simulink model "yixiang"  (R2024a)
settings: Solver=FixedStepDiscrete  StartTime=0.0  StopTime=0.01  FixedStep=1e-8  RelTol=1e-3
libraries: hdlsllib x60, simulink x1
(part 1 of 2)
settings Model: Creator=17862  LastModifiedBy=zyy
settings SolverCC: AlgebraicLoopSolver=TrustRegion  AutoInsertRateTranBlk=on
settings DataIOCC: ReturnWorkspaceOutputs=off
settings OptimizationCC: BlockReduction=off  ConditionallyExecuteInputs=off  DefaultParameterBehavior=Inlined
settings DebuggingCC: AlgebraicLoopMsg=error  SingleTaskRateTransMsg=error  UnconnectedInputMsg=warning  UnconnectedOutputMsg=warning  UnconnectedLineMsg=warning  ArithmeticOperatorsInVariantConditions=warning
settings HardwareCC: ProdBitPerPointer=32  ProdBitPerSizeT=32  ProdBitPerPtrDiffT=32  ProdLargestAtomicFloat=None  ProdIntDivRoundTo=Undefined  ProdEndianess=Unspecified  ProdWordSize=32  ProdHWDeviceType=ASIC/FPGA->ASIC/FPGA  TargetBitPerPointer=64  TargetBitPerSizeT=64  TargetBitPerPtrDiffT=64  TargetLongLongMode=on  TargetIntDivRoundTo=Zero  TargetEndianess=LittleEndian  TargetWordSize=64  TargetHWDeviceType=Custom Processor->MATLAB Host Computer  ProdEqTarget=off
settings ModelReferenceCC: EnableRefExpFcnMdlSchedulingChecks=on
settings SFSimCC: CustomCodeUndefinedFunction=UseInterfaceOnly
settings RTWCC: GPUComputeCapability=3.5

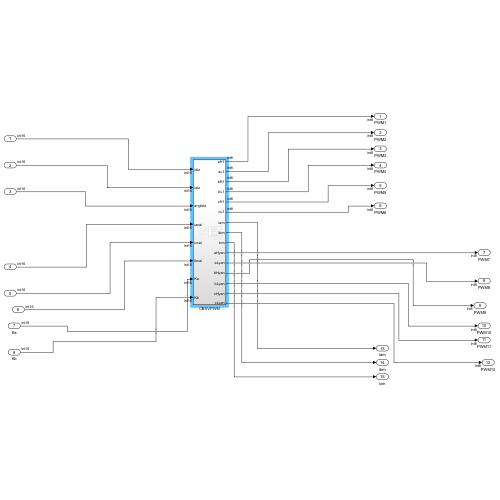
[thumbnail: Simulink's stored preview of the top-level diagram]
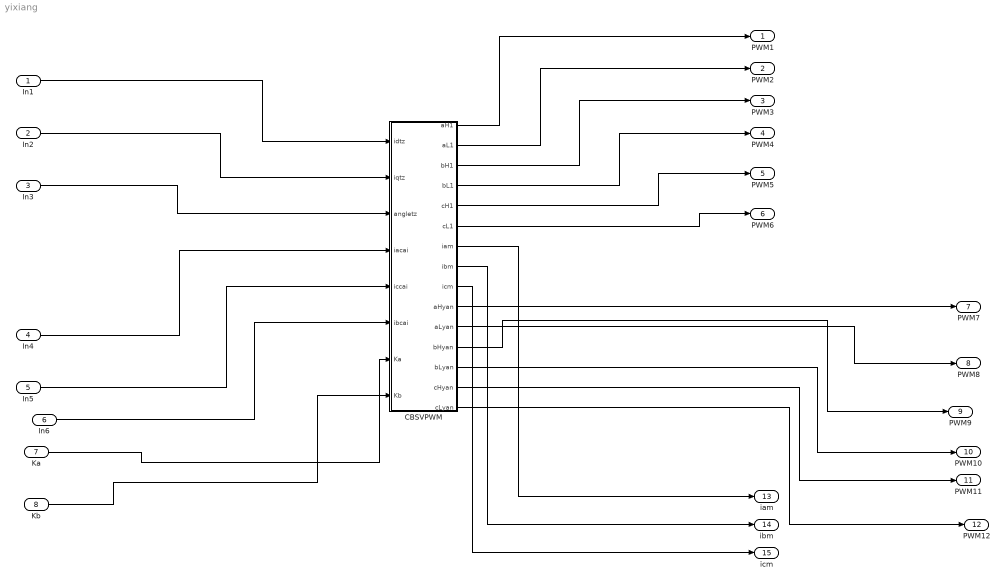
== system yixiang ==
  In1 : Inport  OutDataTypeStr=int16
  In2 : Inport  Port=2  OutDataTypeStr=int16
  In3 : Inport  Port=3  OutDataTypeStr=int16
  In4 : Inport  Port=4  OutDataTypeStr=int16
  In5 : Inport  Port=5  OutDataTypeStr=int16
  In6 : Inport  Port=6  OutDataTypeStr=int16
  Ka : Inport  Port=7  OutDataTypeStr=int16
  Kb : Inport  Port=8  OutDataTypeStr=int16
  CBSVPWM : Subsystem
  PWM1 : Outport  OutDataTypeStr=int8
  PWM2 : Outport  Port=2  OutDataTypeStr=int8
  PWM3 : Outport  Port=3  OutDataTypeStr=int8
  PWM4 : Outport  Port=4  OutDataTypeStr=int8
  PWM5 : Outport  Port=5  OutDataTypeStr=int8
  PWM6 : Outport  Port=6  OutDataTypeStr=int8
  PWM7 : Outport  Port=7  OutDataTypeStr=int8
  PWM8 : Outport  Port=8  OutDataTypeStr=int8
  PWM9 : Outport  Port=9  OutDataTypeStr=int8
  PWM10 : Outport  Port=10  OutDataTypeStr=int8
  PWM11 : Outport  Port=11  OutDataTypeStr=int8
  PWM12 : Outport  Port=12  OutDataTypeStr=int8
  iam : Outport  Port=13
  ibm : Outport  Port=14
  icm : Outport  Port=15
  wires:
  CBSVPWM/12(bHyan) -> PWM9/1
  CBSVPWM/13(bLyan) -> PWM10/1
  CBSVPWM/11(aLyan) -> PWM8/1
  CBSVPWM/15(cLyan) -> PWM12/1
  CBSVPWM/14(cHyan) -> PWM11/1
  CBSVPWM/10(aHyan) -> PWM7/1
  CBSVPWM/6(cL1) -> PWM6/1
  CBSVPWM/5(cH1) -> PWM5/1
  CBSVPWM/2(aL1) -> PWM2/1
  CBSVPWM/1(aH1) -> PWM1/1
  CBSVPWM/3(bH1) -> PWM3/1
  CBSVPWM/4(bL1) -> PWM4/1
  In1/1 -> CBSVPWM/1(idtz)
  In2/1 -> CBSVPWM/2(iqtz)
  In3/1 -> CBSVPWM/3(angletz)
  In4/1 -> CBSVPWM/4(iacai)
  In5/1 -> CBSVPWM/5(iccai)
  In6/1 -> CBSVPWM/6(ibcai)
  CBSVPWM/7(iam) -> iam/1
  CBSVPWM/8(ibm) -> ibm/1
  CBSVPWM/9(icm) -> icm/1
  Ka/1 -> CBSVPWM/7(Ka)
  Kb/1 -> CBSVPWM/8(Kb)

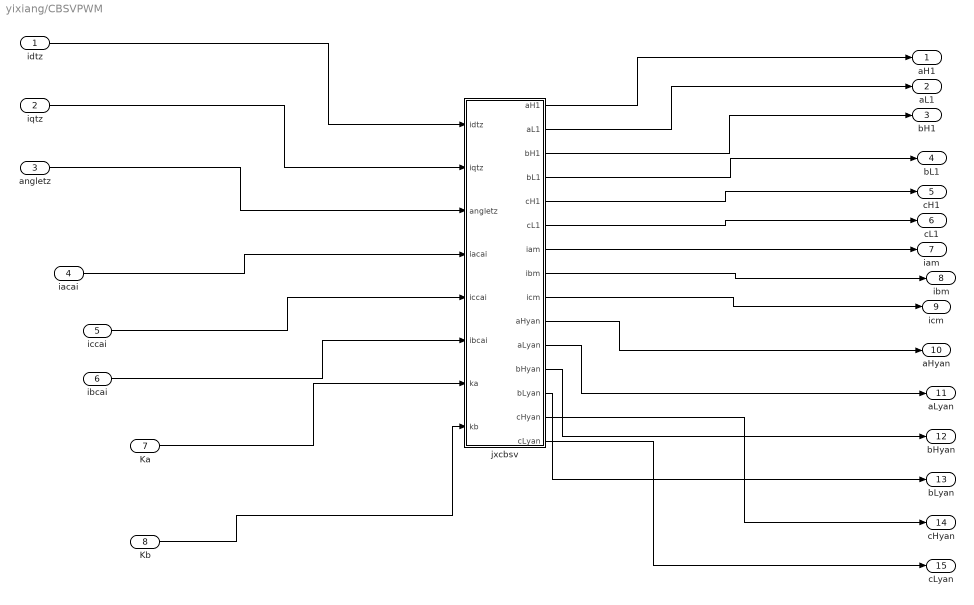
== system yixiang/CBSVPWM ==
  idtz : Inport  OutDataTypeStr=int16
  iqtz : Inport  Port=2  OutDataTypeStr=int16
  angletz : Inport  Port=3  OutDataTypeStr=int16
  iacai : Inport  Port=4  OutDataTypeStr=int16
  iccai : Inport  Port=5  OutDataTypeStr=int16
  ibcai : Inport  Port=6  OutDataTypeStr=int16
  Ka : Inport  Port=7  OutDataTypeStr=int16
  Kb : Inport  Port=8  OutDataTypeStr=int16
  jxcbsv : Subsystem
  aH1 : Outport  OutDataTypeStr=int8
  aL1 : Outport  Port=2  OutDataTypeStr=int8
  bH1 : Outport  Port=3  OutDataTypeStr=int8
  bL1 : Outport  Port=4  OutDataTypeStr=int8
  cH1 : Outport  Port=5  OutDataTypeStr=int8
  cL1 : Outport  Port=6  OutDataTypeStr=int8
  iam : Outport  Port=7
  ibm : Outport  Port=8
  icm : Outport  Port=9
  aHyan : Outport  Port=10
  aLyan : Outport  Port=11
  bHyan : Outport  Port=12
  bLyan : Outport  Port=13
  cHyan : Outport  Port=14
  cLyan : Outport  Port=15
  wires:
  iqtz/1 -> jxcbsv/2(iqtz)
  jxcbsv/6(cL1) -> cL1/1
  jxcbsv/3(bH1) -> bH1/1
  jxcbsv/2(aL1) -> aL1/1
  jxcbsv/4(bL1) -> bL1/1
  iacai/1 -> jxcbsv/4(iacai)
  jxcbsv/5(cH1) -> cH1/1
  jxcbsv/1(aH1) -> aH1/1
  angletz/1 -> jxcbsv/3(angletz)
  idtz/1 -> jxcbsv/1(idtz)
  iccai/1 -> jxcbsv/5(iccai)
  ibcai/1 -> jxcbsv/6(ibcai)
  jxcbsv/7(iam) -> iam/1
  jxcbsv/8(ibm) -> ibm/1
  jxcbsv/9(icm) -> icm/1
  jxcbsv/13(bLyan) -> bLyan/1
  jxcbsv/12(bHyan) -> bHyan/1
  jxcbsv/10(aHyan) -> aHyan/1
  jxcbsv/15(cLyan) -> cLyan/1
  jxcbsv/14(cHyan) -> cHyan/1
  jxcbsv/11(aLyan) -> aLyan/1
  Ka/1 -> jxcbsv/7(ka)
  Kb/1 -> jxcbsv/8(kb)

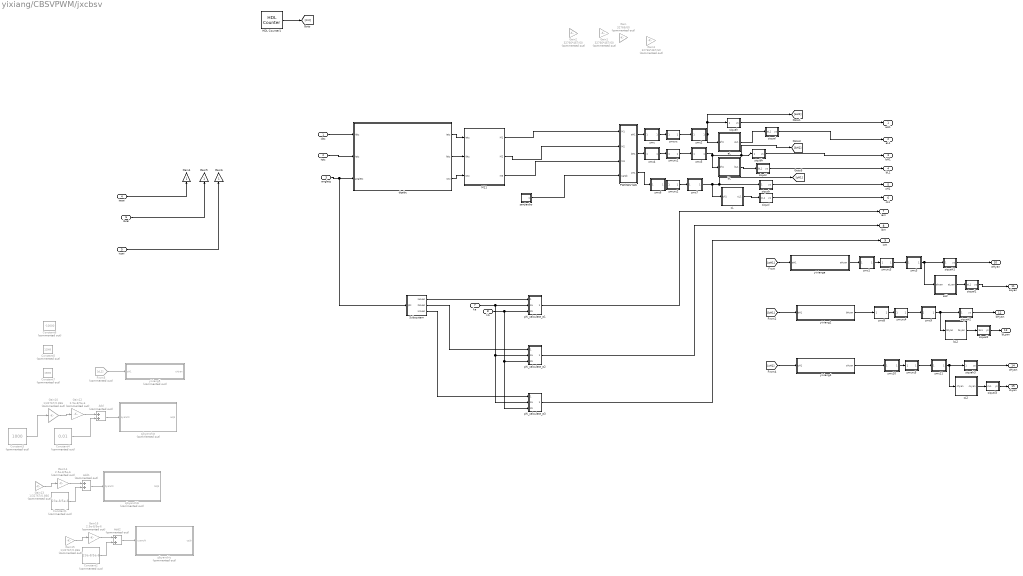
== system yixiang/CBSVPWM/jxcbsv ==
  idtz : Inport  OutDataTypeStr=int16
  iqtz : Inport  Port=2  OutDataTypeStr=int16
  angletz : Inport  Port=3  OutDataTypeStr=int16
  iacai : Inport  Port=4
  iccai : Inport  Port=5
  ibcai : Inport  Port=6
  ka : Inport  Port=7
  kb : Inport  Port=8
  Add : Sum  Commented=on  AccumDataTypeStr=fixdt(1,30,29)
  Add1 : Sum  Commented=on  OutDataTypeStr=fixdt(1,30,29)  AccumDataTypeStr=fixdt(1,30,29)
  Add2 : Sum  Commented=on  OutDataTypeStr=fixdt(1,30,29)  AccumDataTypeStr=fixdt(1,30,29)
  Constant1 : Constant  Commented=on  Value=23e-8/5e-6  OutDataTypeStr=fixdt(1,7,6)  SampleTime=1e-8
  Constant2 : Constant  Commented=on  Value=23e-8/5e-6  OutDataTypeStr=fixdt(1,7,6)  SampleTime=1e-8
  Constant3 : Constant  Commented=on  Value=1000  OutDataTypeStr=int16  SampleTime=1e-8
  Constant4 : Constant  Commented=on  Value=0.01  OutDataTypeStr=fixdt(1,7,6)  SampleTime=1e-8
  Constant5 : Constant  Commented=on  Value=12000  OutDataTypeStr=int16  SampleTime=2e-8
  Constant6 : Constant  Commented=on  Value=-10000  OutDataTypeStr=int16  SampleTime=2e-8
  Constant7 : Constant  Commented=on  Value=15000  OutDataTypeStr=int16  SampleTime=2e-8
  From5 : From  Commented=on  GotoTag=cL1
  Gain : Gain  Commented=on  Gain=32766/60  OutDataTypeStr=int16
  Gain1 : Gain  Commented=on  Gain=32766*4E7/60  OutDataTypeStr=int16
  Gain10 : Gain  Commented=on  Gain=1/32767/0.866  OutDataTypeStr=fixdt(1,21,20)
  Gain12 : Gain  Commented=on  Gain=2.5e-8/5e-6  OutDataTypeStr=fixdt(1,30,29)
  Gain13 : Gain  Commented=on  Gain=1/32767/0.866  OutDataTypeStr=fixdt(1,21,20)
  Gain14 : Gain  Commented=on  Gain=2.5e-8/5e-6  OutDataTypeStr=fixdt(1,30,29)
  Gain15 : Gain  Commented=on  Gain=1/32767/0.866  OutDataTypeStr=fixdt(1,21,20)
  Gain16 : Gain  Commented=on  Gain=2.5e-8/5e-6  OutDataTypeStr=fixdt(1,30,29)
  Gain2 : Gain  Commented=on  Gain=32766*4E7/60  OutDataTypeStr=int16
  Gain3 : Gain  Commented=on  Gain=32766*4E7/60  OutDataTypeStr=int16
  Gain4 : Gain  OutDataTypeStr=int16
  Gain5 : Gain  OutDataTypeStr=int16
  Gain6 : Gain  OutDataTypeStr=int16
  HDL Counter1 : hdlsllib/Sources/HDL Counter  CountType=Count limited  CountInit=0  CountStep=1  CountMax=250  CountFromType=Initial value  CountFrom=0  CountResetPort=off  CountLoadPort=off  CountEnbPort=off  CountDirPort=off  CountHitOutputPort=off  CountDataType=Unsigned  CountWordLen=20  CountFracLen=0  CountSampTime=1/10000/5000
  M11 : Subsystem
  PWMWUYAN : Subsystem
  Subsystem : Subsystem
  aL : Subsystem
  aL2 : Subsystem
  bL : Subsystem
  bL2 : Subsystem
  cL : Subsystem
  cL2 : Subsystem
  dqabc : Subsystem
  phi_calculate_a1 : Subsystem
  phi_calculate_a2 : Subsystem
  phi_calculate_a3 : Subsystem
  sanjiaobo : Subsystem
  siquah : Subsystem
  siquah1 : Subsystem
  siquah2 : Subsystem
  siquah3 : Subsystem
  siqual : Subsystem
  siqual1 : Subsystem
  siqual2 : Subsystem
  siqual3 : Subsystem
  siqubh : Subsystem
  siqubl : Subsystem
  siquch : Subsystem
  siqucl : Subsystem
  sjbyanchia : Subsystem  Commented=on
  sjbyanchib : Subsystem  Commented=on
  sjbyanchic : Subsystem  Commented=on
  yixiang2 : Subsystem
  yixiang4 : Subsystem
  yixiang5 : Subsystem  Commented=on
  yixianga : Subsystem
  zmc : Subsystem
  zmc1 : Subsystem
  zmc10 : Subsystem
  zmc11 : Subsystem
  zmc2 : Subsystem
  zmc3 : Subsystem
  zmc4 : Subsystem
  zmc5 : Subsystem
  zmc6 : Subsystem
  zmc7 : Subsystem
  zmc8 : Subsystem
  zmc9 : Subsystem
  zmcxc : Subsystem
  zmcxc1 : Subsystem
  zmcxc2 : Subsystem
  zmcxc3 : Subsystem
  zmcxc4 : Subsystem
  zmcxc5 : Subsystem
  aH1 : Outport  OutDataTypeStr=int8
  aL1 : Outport  Port=2  OutDataTypeStr=int8
  bH1 : Outport  Port=3  OutDataTypeStr=int8
  bL1 : Outport  Port=4  OutDataTypeStr=int8
  cH1 : Outport  Port=5  OutDataTypeStr=int8
  cL1 : Outport  Port=6  OutDataTypeStr=int8
  iam : Outport  Port=7
  ibm : Outport  Port=8
  icm : Outport  Port=9
  aHyan : Outport  Port=10  OutDataTypeStr=int8
  aLyan : Outport  Port=11  OutDataTypeStr=int8
  bHyan : Outport  Port=12  OutDataTypeStr=int8
  bLyan : Outport  Port=13  OutDataTypeStr=int8
  cHyan : Outport  Port=14  OutDataTypeStr=int8
  cLyan : Outport  Port=15  OutDataTypeStr=int8
  wires:
  iqtz/1 -> dqabc/2(iqtz)
  idtz/1 -> dqabc/1(idtz)
  dqabc/1(iatz) -> M11/1(iatz)
  dqabc/2(ibtz) -> M11/2(ibtz)
  dqabc/3(ictz) -> M11/3(ictz)
  Add/1 -> sjbyanchia/1(ayanchi)
  Gain12/1 -> Add/1
  Gain10/1 -> Gain12/1
  sanjiaobo/1(sanjb) -> PWMWUYAN/4(sanjb)
  Add2/1 -> sjbyanchic/1(cyanchi)
  Gain15/1 -> Gain16/1
  Gain16/1 -> Add2/1
  Constant2/1 -> Add2/2
  Add1/1 -> sjbyanchib/1(byanchi)
  Gain13/1 -> Gain14/1
  Gain14/1 -> Add1/1
  Constant1/1 -> Add1/2
  Constant4/1 -> Add/2
  Constant3/1 -> Gain10/1
  HDL Counter1/1 -> [cnt]
  M11/2(M2) -> PWMWUYAN/2(M2)
  M11/3(M3) -> PWMWUYAN/3(M3)
  M11/1(M1) -> PWMWUYAN/1(M1)
  PWMWUYAN/1(aH1) -> zmc/1(aH1)
  zmc/1(bH1) -> zmcxc/1(bH1)
  zmcxc/1(aL1) -> zmc2/1(aH1)
  zmc2/1(bH1) -> siquah/1(aH1), [aH1], aL/1(ah1)
  zmc4/1(bH1) -> zmcxc1/1(bH1)
  zmcxc1/1(aL1) -> zmc5/1(aH1)
  aL/1(aL1) -> siqual/1(aL1)
  PWMWUYAN/2(bH1) -> zmc4/1(aH1)
  zmc5/1(bH1) -> bL/1(bh1), [bH1], siqubh/1(bH1)
  bL/1(bL1) -> siqubl/1(bL1)
  zmc6/1(bH1) -> zmcxc2/1(bH1)
  zmcxc2/1(aL1) -> zmc7/1(aH1)
  PWMWUYAN/3(cH1) -> zmc6/1(aH1)
  zmc7/1(bH1) -> [cH1], siquch/1(cH1), cL/1(ch1)
  cL/1(cL1) -> siqucl/1(cL1)
  siqubl/1(ys) -> bL1/1
  siquah/1(ys) -> aH1/1
  siqubh/1(ys) -> bH1/1
  siquch/1(ys) -> cH1/1
  siqucl/1(ys) -> cL1/1
  iacai/1 -> Gain4/1
  ibcai/1 -> Gain5/1
  iccai/1 -> Gain6/1
  phi_calculate_a1/1(iam) -> iam/1
  angletz/1 -> Subsystem/1(phi), dqabc/3(angletz)
  Subsystem/1(iasuan) -> phi_calculate_a1/1(iacai)
  ka/1 -> phi_calculate_a3/2(ka), phi_calculate_a2/2(ka), phi_calculate_a1/2(ka)
  kb/1 -> phi_calculate_a3/3(kb), phi_calculate_a2/3(kb), phi_calculate_a1/3(kb)
  siqual/1(ys) -> aL1/1
  [aH1] -> yixianga/1(aH1)
  [bH1] -> yixiang2/1(bH1)
  [cH1] -> yixiang4/1(cH1)
  From5/1 -> yixiang5/1(cH1)
  Subsystem/2(ibsuan) -> phi_calculate_a2/1(ibcai)
  Subsystem/3(icsuan) -> phi_calculate_a3/1(iccai)
  phi_calculate_a2/1(ibm) -> ibm/1
  phi_calculate_a3/1(icm) -> icm/1
  aL2/1(aLyan) -> siqual1/1(aL1)
  yixianga/1(aHyan) -> zmc1/1(aH1)
  zmc3/1(bH1) -> aL2/1(ahyan), siquah1/1(aH1)
  zmcxc3/1(aL1) -> zmc3/1(aH1)
  zmc1/1(bH1) -> zmcxc3/1(bH1)
  zmcxc4/1(aL1) -> zmc9/1(aH1)
  yixiang2/1(bHyan) -> zmc8/1(aH1)
  zmc8/1(bH1) -> zmcxc4/1(bH1)
  zmc9/1(bH1) -> bL2/1(bhyan), siquah2/1(bH1)
  siqual1/1(ys) -> aLyan/1
  siquah1/1(ys) -> aHyan/1
  siquah2/1(ys) -> bHyan/1
  siqual2/1(ys) -> bLyan/1
  bL2/1(bLyan) -> siqual2/1(bL1)
  zmc10/1(bH1) -> zmcxc5/1(bH1)
  zmcxc5/1(aL1) -> zmc11/1(aH1)
  yixiang4/1(cHyan) -> zmc10/1(aH1)
  zmc11/1(bH1) -> cL2/1(chyan), siquah3/1(cH1)
  cL2/1(cLyan) -> siqual3/1(cL1)
  siquah3/1(ys) -> cHyan/1
  siqual3/1(ys) -> cLyan/1

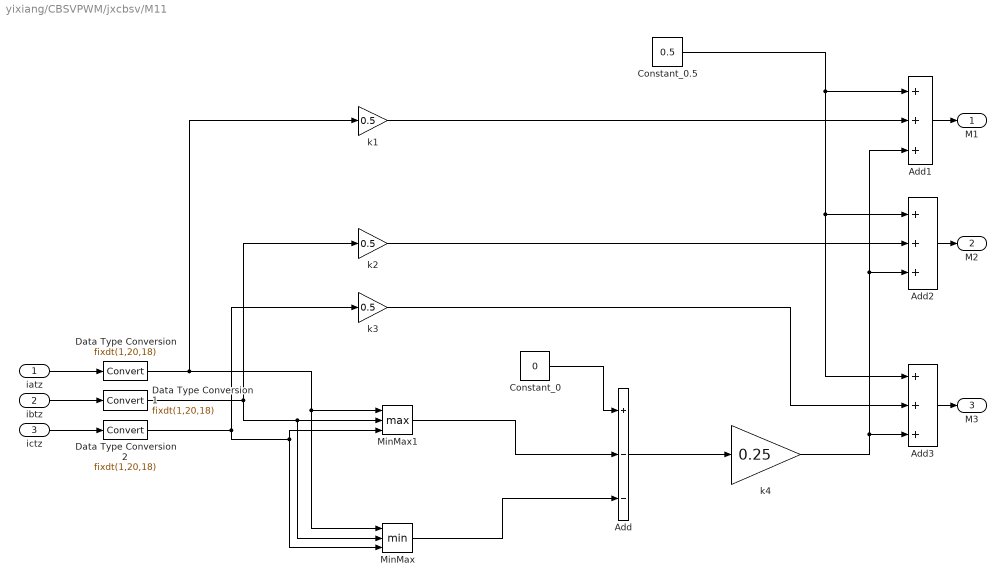
== system yixiang/CBSVPWM/jxcbsv/M11 ==
  iatz : Inport
  ibtz : Inport  Port=2
  ictz : Inport  Port=3
  Add : Sum  Inputs=+--  OutDataTypeStr=fixdt(1,20,18)
  Add1 : Sum  Inputs=+++  OutDataTypeStr=fixdt(1,20,18)  AccumDataTypeStr=fixdt(1,20,18)
  Add2 : Sum  Inputs=+++  OutDataTypeStr=fixdt(1,20,18)  AccumDataTypeStr=fixdt(1,20,18)
  Add3 : Sum  Inputs=+++  OutDataTypeStr=fixdt(1,20,18)  AccumDataTypeStr=fixdt(1,20,18)
  Constant_0 : Constant  Value=0  OutDataTypeStr=fixdt(1,20,18)  SampleTime=2e-8
  Constant_0.5 : Constant  Value=0.5  OutDataTypeStr=fixdt(1,20,18)  SampleTime=2e-8
  Data Type Conversion : DataTypeConversion  OutDataTypeStr=fixdt(1,20,18)  SaturateOnIntegerOverflow=off  RndMeth=Floor
  Data Type Conversion1 : DataTypeConversion  OutDataTypeStr=fixdt(1,20,18)  SaturateOnIntegerOverflow=off  RndMeth=Floor
  Data Type Conversion2 : DataTypeConversion  OutDataTypeStr=fixdt(1,20,18)  SaturateOnIntegerOverflow=off  RndMeth=Floor
  MinMax : MinMax  Inputs=3
  MinMax1 : MinMax  Function=max  Inputs=3
  k1 : Gain  Gain=0.5  OutDataTypeStr=fixdt(1,20,18)
  k2 : Gain  Gain=0.5  OutDataTypeStr=fixdt(1,20,18)
  k3 : Gain  Gain=0.5  OutDataTypeStr=fixdt(1,20,18)
  k4 : Gain  Gain=0.25  OutDataTypeStr=fixdt(1,20,18)
  M1 : Outport  VectorParamsAs1DForOutWhenUnconnected=off
  M2 : Outport  Port=2  VectorParamsAs1DForOutWhenUnconnected=off
  M3 : Outport  Port=3  VectorParamsAs1DForOutWhenUnconnected=off
  wires:
  Constant_0/1 -> Add/1
  Add/1 -> k4/1
  MinMax1/1 -> Add/2
  Add1/1 -> M1/1
  Add2/1 -> M2/1
  Add3/1 -> M3/1
  Constant_0.5/1 -> Add3/1, Add2/1, Add1/1
  k1/1 -> Add1/2
  k4/1 -> Add1/3, Add2/3, Add3/3
  k2/1 -> Add2/2
  k3/1 -> Add3/2
  ibtz/1 -> Data Type Conversion1/1
  ictz/1 -> Data Type Conversion2/1
  MinMax/1 -> Add/3
  iatz/1 -> Data Type Conversion/1
  Data Type Conversion1/1 -> k2/1, MinMax1/2, MinMax/2
  Data Type Conversion2/1 -> k3/1, MinMax1/3, MinMax/3
  Data Type Conversion/1 -> MinMax1/1, MinMax/1, k1/1

== system yixiang/CBSVPWM/jxcbsv/PWMWUYAN ==
  M1 : Inport
  M2 : Inport  Port=2
  M3 : Inport  Port=3
  sanjb : Inport  Port=4
  Add : Sum  Inputs=+-
  Add2 : Sum  Inputs=+-
  Add4 : Sum  Inputs=+-
  Relay : Relay  OnSwitchValue=0  OffSwitchValue=0  OutDataTypeStr=int8
  Relay1 : Relay  OnSwitchValue=0  OffSwitchValue=0  OutDataTypeStr=int8
  Relay2 : Relay  OnSwitchValue=0  OffSwitchValue=0  OutDataTypeStr=int8
  aH1 : Outport  VectorParamsAs1DForOutWhenUnconnected=off
  bH1 : Outport  Port=2  VectorParamsAs1DForOutWhenUnconnected=off
  cH1 : Outport  Port=3  VectorParamsAs1DForOutWhenUnconnected=off
  wires:
  M1/1 -> Add/1
  M3/1 -> Add4/1
  M2/1 -> Add2/1
  Add/1 -> Relay/1
  Add4/1 -> Relay2/1
  Add2/1 -> Relay1/1
  sanjb/1 -> Add4/2, Add2/2, Add/2
  Relay/1 -> aH1/1
  Relay1/1 -> bH1/1
  Relay2/1 -> cH1/1

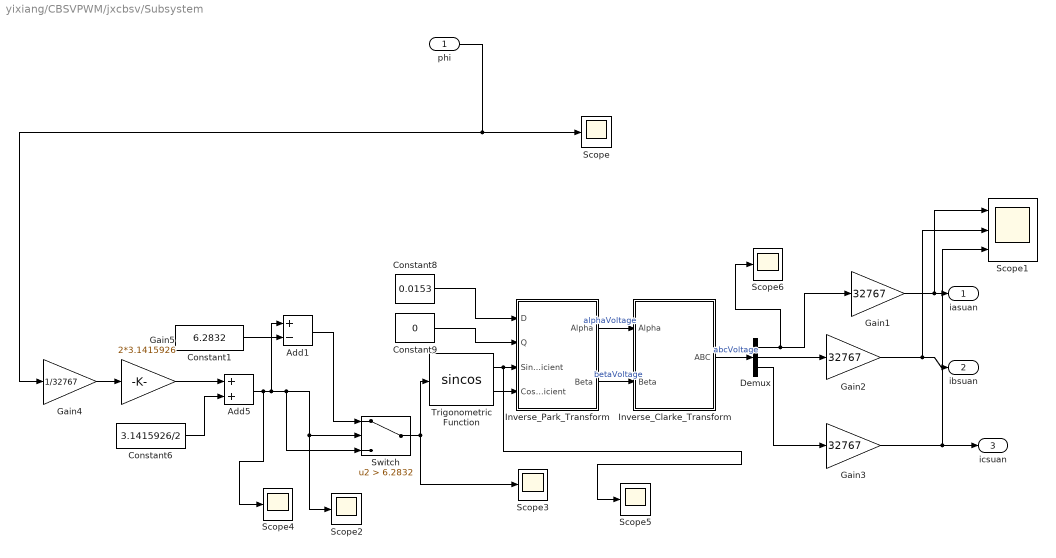
== system yixiang/CBSVPWM/jxcbsv/Subsystem ==
  phi : Inport
  Add1 : Sum  Inputs=+-  OutDataTypeStr=fixdt(1,16,10)  AccumDataTypeStr=fixdt(1,16,10)
  Add5 : Sum  OutDataTypeStr=fixdt(1,16,10)  AccumDataTypeStr=fixdt(1,16,10)
  Constant1 : Constant  Value=6.2832  OutDataTypeStr=fixdt(1,16,10)  SampleTime=2e-8
  Constant6 : Constant  Value=3.1415926/2  OutDataTypeStr=fixdt(1,16,10)  SampleTime=2e-8
  Constant8 : Constant  Value=0.0153  OutDataTypeStr=fixdt(1,32,27)  SampleTime=2e-8
  Constant9 : Constant  Value=0  OutDataTypeStr=uint16  SampleTime=2e-8
  Demux : Demux  Outputs=3
  Gain1 : Gain  Gain=32767  OutDataTypeStr=int16
  Gain2 : Gain  Gain=32767  OutDataTypeStr=int16
  Gain3 : Gain  Gain=32767  OutDataTypeStr=int16
  Gain4 : Gain  Gain=1/32767  OutDataTypeStr=fixdt(1,16,10)
  Gain5 : Gain  Gain=2*3.1415926  OutDataTypeStr=fixdt(1,16,10)
  Inverse_Clarke_Transform : Subsystem  VariantControl=INVERSE_CLARKE_TRANSFORM
      mask Display:
      | port_label('input',1,'\alpha','texmode', 'on')
      | port_label('input',2,'\beta','texmode', 'on')
      | port_label('output',1,'ABC')
  Inverse_Park_Transform : Subsystem
      mask Display:
      | port_label('input',1,'D')
      | port_label('input',2,'Q')
      | port_label('input',3,'Sin')
      | port_label('input',4,'Cos')
      | port_label('output',1,'\alpha','texmode', 'on')
      | port_label('output',2,'\beta','texmode', 'on')
  Scope{,2..6} (6 alike) : Scope
  Scope1 : Scope  NumInputPorts=3
  Switch : Switch  Criteria=u2 > Threshold  Threshold=6.2832  OutDataTypeStr=fixdt(1,16,10)  SaturateOnIntegerOverflow=off  InputSameDT=off
  Trigonometric Function : Trigonometry  Operator=sincos  ApproximationMethod=CORDIC  NumberOfIterations=16
  iasuan : Outport
  ibsuan : Outport  Port=2
  icsuan : Outport  Port=3
  wires:
  Inverse_Park_Transform/1(Alpha) -> Inverse_Clarke_Transform/1(Alpha)  "alphaVoltage"
  Inverse_Clarke_Transform/1(ABC) -> Demux/1  "abcVoltage"
  Inverse_Park_Transform/2(Beta) -> Inverse_Clarke_Transform/2(Beta)  "betaVoltage"
  Constant8/1 -> Inverse_Park_Transform/1(D)
  Constant9/1 -> Inverse_Park_Transform/2(Q)
  Gain4/1 -> Gain5/1
  Trigonometric Function/1 -> Scope5/1, Inverse_Park_Transform/3(Sin_Coefficient)
  Trigonometric Function/2 -> Inverse_Park_Transform/4(Cos_Coefficient)
  Demux/3 -> Gain3/1
  phi/1 -> Scope/1, Gain4/1
  Demux/1 -> Scope6/1, Gain1/1
  Demux/2 -> Gain2/1
  Gain5/1 -> Add5/1
  Add5/1 -> Scope4/1, Add1/1, Switch/3, Scope2/1, Switch/2
  Constant6/1 -> Add5/2
  Gain1/1 -> Scope1/1, iasuan/1
  Gain2/1 -> Scope1/2, ibsuan/1
  Gain3/1 -> Scope1/3, icsuan/1
  Switch/1 -> Trigonometric Function/1, Scope3/1
  Add1/1 -> Switch/1
  Constant1/1 -> Add1/2

== system yixiang/CBSVPWM/jxcbsv/aL ==
  ah1 : Inport
  Data Type Conversion : DataTypeConversion  OutDataTypeStr=boolean  SaturateOnIntegerOverflow=off  RndMeth=Floor
  Data Type Conversion1 : DataTypeConversion  OutDataTypeStr=int8  SaturateOnIntegerOverflow=off  RndMeth=Floor
  Logical Operator : Logic  Operator=NOT  AllPortsSameDT=off  OutDataTypeStr=boolean
  aL1 : Outport  VectorParamsAs1DForOutWhenUnconnected=off
  wires:
  Logical Operator/1 -> Data Type Conversion1/1
  ah1/1 -> Data Type Conversion/1
  Data Type Conversion/1 -> Logical Operator/1
  Data Type Conversion1/1 -> aL1/1

== system yixiang/CBSVPWM/jxcbsv/aL2 ==
  ahyan : Inport
  Data Type Conversion : DataTypeConversion  OutDataTypeStr=boolean  SaturateOnIntegerOverflow=off  RndMeth=Floor
  Data Type Conversion1 : DataTypeConversion  OutDataTypeStr=int8  SaturateOnIntegerOverflow=off  RndMeth=Floor
  Logical Operator : Logic  Operator=NOT  AllPortsSameDT=off  OutDataTypeStr=boolean
  aLyan : Outport  VectorParamsAs1DForOutWhenUnconnected=off
  wires:
  Logical Operator/1 -> Data Type Conversion1/1
  ahyan/1 -> Data Type Conversion/1
  Data Type Conversion/1 -> Logical Operator/1
  Data Type Conversion1/1 -> aLyan/1

== system yixiang/CBSVPWM/jxcbsv/bL ==
  bh1 : Inport
  Data Type Conversion : DataTypeConversion  OutDataTypeStr=boolean  SaturateOnIntegerOverflow=off  RndMeth=Floor
  Data Type Conversion1 : DataTypeConversion  OutDataTypeStr=int8  SaturateOnIntegerOverflow=off  RndMeth=Floor
  Logical Operator : Logic  Operator=NOT  AllPortsSameDT=off  OutDataTypeStr=boolean
  bL1 : Outport  VectorParamsAs1DForOutWhenUnconnected=off
  wires:
  Data Type Conversion1/1 -> bL1/1
  Logical Operator/1 -> Data Type Conversion1/1
  bh1/1 -> Data Type Conversion/1
  Data Type Conversion/1 -> Logical Operator/1

== system yixiang/CBSVPWM/jxcbsv/bL2 ==
  bhyan : Inport
  Data Type Conversion : DataTypeConversion  OutDataTypeStr=boolean  SaturateOnIntegerOverflow=off  RndMeth=Floor
  Data Type Conversion1 : DataTypeConversion  OutDataTypeStr=int8  SaturateOnIntegerOverflow=off  RndMeth=Floor
  Logical Operator : Logic  Operator=NOT  AllPortsSameDT=off  OutDataTypeStr=boolean
  bLyan : Outport  VectorParamsAs1DForOutWhenUnconnected=off
  wires:
  Logical Operator/1 -> Data Type Conversion1/1
  bhyan/1 -> Data Type Conversion/1
  Data Type Conversion/1 -> Logical Operator/1
  Data Type Conversion1/1 -> bLyan/1

== system yixiang/CBSVPWM/jxcbsv/cL ==
  ch1 : Inport
  Data Type Conversion : DataTypeConversion  OutDataTypeStr=boolean  SaturateOnIntegerOverflow=off  RndMeth=Floor
  Data Type Conversion1 : DataTypeConversion  OutDataTypeStr=int8  SaturateOnIntegerOverflow=off  RndMeth=Floor
  Logical Operator : Logic  Operator=NOT  AllPortsSameDT=off  OutDataTypeStr=boolean
  cL1 : Outport  VectorParamsAs1DForOutWhenUnconnected=off
  wires:
  Data Type Conversion1/1 -> cL1/1
  Logical Operator/1 -> Data Type Conversion1/1
  ch1/1 -> Data Type Conversion/1
  Data Type Conversion/1 -> Logical Operator/1

== system yixiang/CBSVPWM/jxcbsv/cL2 ==
  chyan : Inport
  Data Type Conversion : DataTypeConversion  OutDataTypeStr=boolean  SaturateOnIntegerOverflow=off  RndMeth=Floor
  Data Type Conversion1 : DataTypeConversion  OutDataTypeStr=int8  SaturateOnIntegerOverflow=off  RndMeth=Floor
  Logical Operator : Logic  Operator=NOT  AllPortsSameDT=off  OutDataTypeStr=boolean
  cLyan : Outport  VectorParamsAs1DForOutWhenUnconnected=off
  wires:
  Logical Operator/1 -> Data Type Conversion1/1
  chyan/1 -> Data Type Conversion/1
  Data Type Conversion/1 -> Logical Operator/1
  Data Type Conversion1/1 -> cLyan/1

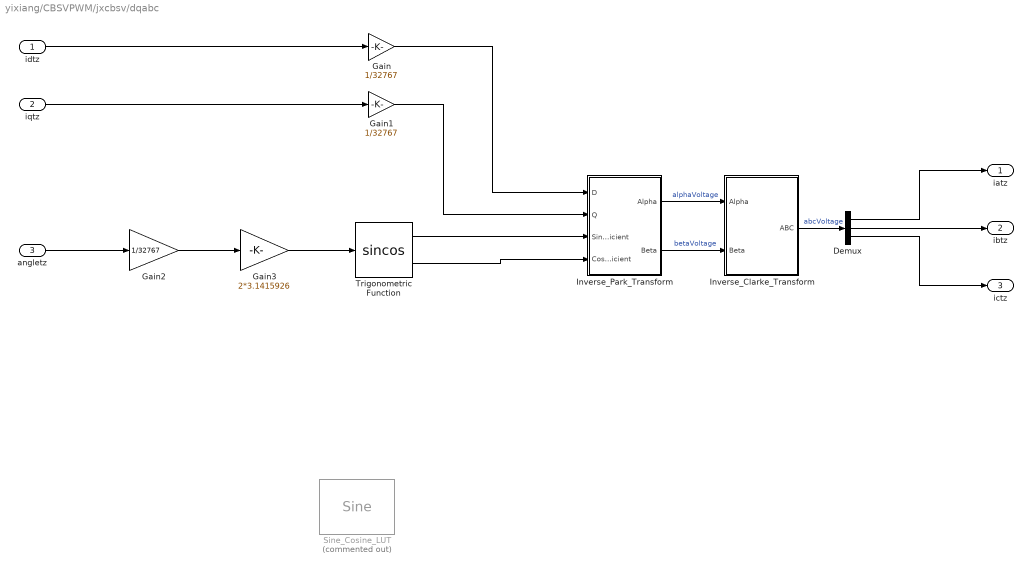
== system yixiang/CBSVPWM/jxcbsv/dqabc ==
  idtz : Inport
  iqtz : Inport  Port=2
  angletz : Inport  Port=3
  Demux : Demux  Outputs=3
  Gain : Gain  Gain=1/32767  OutDataTypeStr=fixdt(1,32,27)
  Gain1 : Gain  Gain=1/32767  OutDataTypeStr=fixdt(1,32,27)
  Gain2 : Gain  Gain=1/32767  OutDataTypeStr=fixdt(1,16,10)
  Gain3 : Gain  Gain=2*3.1415926  OutDataTypeStr=fixdt(1,16,10)
  Inverse_Clarke_Transform : Subsystem  VariantControl=INVERSE_CLARKE_TRANSFORM
      mask Display:
      | port_label('input',1,'\alpha','texmode', 'on')
      | port_label('input',2,'\beta','texmode', 'on')
      | port_label('output',1,'ABC')
  Inverse_Park_Transform : Subsystem
      mask Display:
      | port_label('input',1,'D')
      | port_label('input',2,'Q')
      | port_label('input',3,'Sin')
      | port_label('input',4,'Cos')
      | port_label('output',1,'\alpha','texmode', 'on')
      | port_label('output',2,'\beta','texmode', 'on')
  Sine_Cosine_LUT : simulink/Lookup Tables/Sine  Commented=on  Formula=sin(2*pi*u) and cos(2*pi*u)  NumDataPoints=(2^5)+1  OutputWordLength=32  InternalRulePriority=Speed
  Trigonometric Function : Trigonometry  Operator=sincos  ApproximationMethod=CORDIC  NumberOfIterations=16
  iatz : Outport
  ibtz : Outport  Port=2
  ictz : Outport  Port=3
  wires:
  Gain1/1 -> Inverse_Park_Transform/2(Q)
  Gain/1 -> Inverse_Park_Transform/1(D)
  Inverse_Park_Transform/2(Beta) -> Inverse_Clarke_Transform/2(Beta)  "betaVoltage"
  Inverse_Clarke_Transform/1(ABC) -> Demux/1  "abcVoltage"
  Inverse_Park_Transform/1(Alpha) -> Inverse_Clarke_Transform/1(Alpha)  "alphaVoltage"
  idtz/1 -> Gain/1
  angletz/1 -> Gain2/1
  iqtz/1 -> Gain1/1
  Demux/2 -> ibtz/1
  Demux/1 -> iatz/1
  Trigonometric Function/1 -> Inverse_Park_Transform/3(Sin_Coefficient)
  Trigonometric Function/2 -> Inverse_Park_Transform/4(Cos_Coefficient)
  Gain3/1 -> Trigonometric Function/1
  Gain2/1 -> Gain3/1
  Demux/3 -> ictz/1

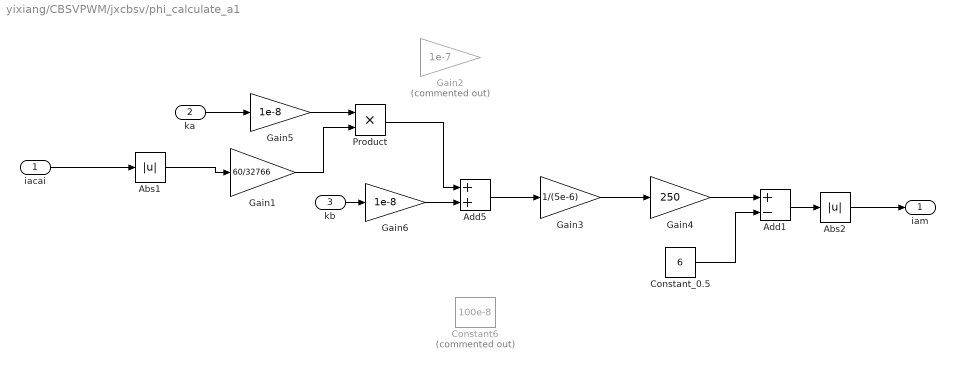
== system yixiang/CBSVPWM/jxcbsv/phi_calculate_a1 ==
  iacai : Inport
  ka : Inport  Port=2
  kb : Inport  Port=3
  Abs1 : Abs  OutDataTypeStr=uint16  SaturateOnIntegerOverflow=off
  Abs2 : Abs  OutDataTypeStr=int16  SaturateOnIntegerOverflow=off
  Add1 : Sum  Inputs=+-  OutDataTypeStr=int16  AccumDataTypeStr=int16
  Add5 : Sum  OutDataTypeStr=fixdt(0,64,40)  AccumDataTypeStr=fixdt(0,64,40)
  Constant6 : Constant  Commented=on  Value=100e-8  OutDataTypeStr=fixdt(0,64,40)  SampleTime=2e-8
  Constant_0.5 : Constant  Value=6  OutDataTypeStr=int16  SampleTime=2e-8
  Gain1 : Gain  Gain=60/32766  OutDataTypeStr=fixdt(0,64,40)
  Gain2 : Gain  Commented=on  Gain=1e-7  OutDataTypeStr=fixdt(0,64,40)
  Gain3 : Gain  Gain=1/(5e-6)  OutDataTypeStr=fixdt(0,64,40)
  Gain4 : Gain  Gain=250  OutDataTypeStr=int16
  Gain5 : Gain  Gain=1e-8  OutDataTypeStr=fixdt(0,64,40)
  Gain6 : Gain  Gain=1e-8  OutDataTypeStr=fixdt(0,64,40)
  Product : Product  OutDataTypeStr=fixdt(0,64,40)
  iam : Outport
  wires:
  Add5/1 -> Gain3/1
  Gain3/1 -> Gain4/1
  iacai/1 -> Abs1/1
  Abs1/1 -> Gain1/1
  Gain4/1 -> Add1/1
  Product/1 -> Add5/1
  Gain1/1 -> Product/2
  ka/1 -> Gain5/1
  kb/1 -> Gain6/1
  Gain5/1 -> Product/1
  Gain6/1 -> Add5/2
  Add1/1 -> Abs2/1
  Abs2/1 -> iam/1
  Constant_0.5/1 -> Add1/2

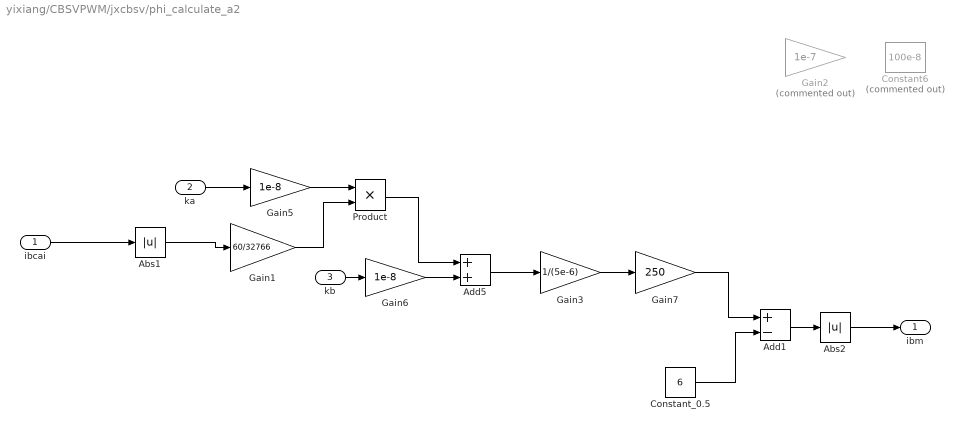
== system yixiang/CBSVPWM/jxcbsv/phi_calculate_a2 ==
  ibcai : Inport
  ka : Inport  Port=2
  kb : Inport  Port=3
  Abs1 : Abs  OutDataTypeStr=uint16  SaturateOnIntegerOverflow=off
  Abs2 : Abs  OutDataTypeStr=int16  SaturateOnIntegerOverflow=off
  Add1 : Sum  Inputs=+-  OutDataTypeStr=int16  AccumDataTypeStr=int16
  Add5 : Sum  OutDataTypeStr=fixdt(0,64,40)  AccumDataTypeStr=fixdt(0,64,40)
  Constant6 : Constant  Commented=on  Value=100e-8  OutDataTypeStr=fixdt(0,64,40)  SampleTime=2e-8
  Constant_0.5 : Constant  Value=6  OutDataTypeStr=int16  SampleTime=2e-8
  Gain1 : Gain  Gain=60/32766  OutDataTypeStr=fixdt(0,64,40)
  Gain2 : Gain  Commented=on  Gain=1e-7  OutDataTypeStr=fixdt(0,64,40)
  Gain3 : Gain  Gain=1/(5e-6)  OutDataTypeStr=fixdt(0,64,40)
  Gain5 : Gain  Gain=1e-8  OutDataTypeStr=fixdt(0,64,40)
  Gain6 : Gain  Gain=1e-8  OutDataTypeStr=fixdt(0,64,40)
  Gain7 : Gain  Gain=250  OutDataTypeStr=int16
  Product : Product  OutDataTypeStr=fixdt(0,64,40)
  ibm : Outport
  wires:
  Add5/1 -> Gain3/1
  Gain3/1 -> Gain7/1
  ibcai/1 -> Abs1/1
  Abs1/1 -> Gain1/1
  Abs2/1 -> ibm/1
  Product/1 -> Add5/1
  Gain1/1 -> Product/2
  ka/1 -> Gain5/1
  kb/1 -> Gain6/1
  Gain5/1 -> Product/1
  Gain6/1 -> Add5/2
  Add1/1 -> Abs2/1
  Gain7/1 -> Add1/1
  Constant_0.5/1 -> Add1/2

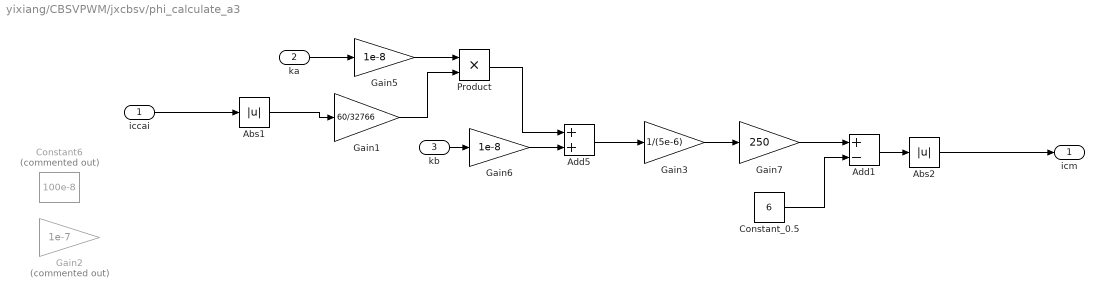
== system yixiang/CBSVPWM/jxcbsv/phi_calculate_a3 ==
  iccai : Inport
  ka : Inport  Port=2
  kb : Inport  Port=3
  Abs1 : Abs  OutDataTypeStr=uint16  SaturateOnIntegerOverflow=off
  Abs2 : Abs  OutDataTypeStr=int16  SaturateOnIntegerOverflow=off
  Add1 : Sum  Inputs=+-  OutDataTypeStr=int16  AccumDataTypeStr=int16
  Add5 : Sum  OutDataTypeStr=fixdt(0,64,40)  AccumDataTypeStr=fixdt(0,64,40)
  Constant6 : Constant  Commented=on  Value=100e-8  OutDataTypeStr=fixdt(0,64,40)  SampleTime=2e-8
  Constant_0.5 : Constant  Value=6  OutDataTypeStr=int16  SampleTime=2e-8
  Gain1 : Gain  Gain=60/32766  OutDataTypeStr=fixdt(0,64,40)
  Gain2 : Gain  Commented=on  Gain=1e-7  OutDataTypeStr=fixdt(0,64,40)
  Gain3 : Gain  Gain=1/(5e-6)  OutDataTypeStr=fixdt(0,64,40)
  Gain5 : Gain  Gain=1e-8  OutDataTypeStr=fixdt(0,64,40)
  Gain6 : Gain  Gain=1e-8  OutDataTypeStr=fixdt(0,64,40)
  Gain7 : Gain  Gain=250  OutDataTypeStr=int16
  Product : Product  OutDataTypeStr=fixdt(0,64,40)
  icm : Outport
  wires:
  Add5/1 -> Gain3/1
  iccai/1 -> Abs1/1
  Abs1/1 -> Gain1/1
  Product/1 -> Add5/1
  Gain1/1 -> Product/2
  ka/1 -> Gain5/1
  kb/1 -> Gain6/1
  Gain5/1 -> Product/1
  Gain6/1 -> Add5/2
  Add1/1 -> Abs2/1
  Gain7/1 -> Add1/1
  Abs2/1 -> icm/1
  Constant_0.5/1 -> Add1/2
  Gain3/1 -> Gain7/1

== system yixiang/CBSVPWM/jxcbsv/sanjiaobo ==
  Abs1 : Abs  OutDataTypeStr=fixdt(1,32,30)  SaturateOnIntegerOverflow=off
  Add : Sum  Commented=on  Inputs=+-
  Add5 : Sum  Inputs=+-  OutDataTypeStr=fixdt(1,32,30)  AccumDataTypeStr=fixdt(1,32,30)
  Constant : Constant  Commented=on  Value=125  OutDataTypeStr=fixdt(1,20,0)  SampleTime=2e-8
  Constant1 : Constant  Commented=on  Value=250  OutDataTypeStr=fixdt(1,20,0)  SampleTime=2e-8
  Constant6 : Constant  Value=0.5  OutDataTypeStr=fixdt(1,32,30)  SampleTime=2e-8
  Gain : Gain  Commented=on  Gain=1/125  OutDataTypeStr=fixdt(1,20,18)
  Gain2 : Gain  Gain=1/250  OutDataTypeStr=fixdt(1,32,30)
  Gain3 : Gain  Gain=2  OutDataTypeStr=fixdt(1,32,30)
  HDL Counter1 : hdlsllib/Sources/HDL Counter  Commented=on  CountType=Count limited  CountInit=0  CountStep=1  CountMax=250  CountFromType=Initial value  CountFrom=0  CountResetPort=off  CountLoadPort=off  CountEnbPort=off  CountDirPort=off  CountHitOutputPort=off  CountDataType=Unsigned  CountWordLen=20  CountFracLen=0  CountSampTime=1/10000/5000
  HDL Counter2 : hdlsllib/Sources/HDL Counter  CountType=Count limited  CountInit=0  CountStep=1  CountMax=250  CountFromType=Initial value  CountFrom=0  CountResetPort=off  CountLoadPort=off  CountEnbPort=off  CountDirPort=off  CountHitOutputPort=off  CountDataType=Unsigned  CountWordLen=20  CountFracLen=0  CountSampTime=1/10000/5000
  Multiport Switch : MultiPortSwitch  Commented=on  DataPortOrder=Zero-based contiguous  Inputs=2  zeroidx=on  OutDataTypeStr=fixdt(1,20,0)  SaturateOnIntegerOverflow=off  InputSameDT=off
  Relational Operator : RelationalOperator  Commented=on  Operator=<=  OutDataTypeStr=boolean  InputSameDT=off
  sanjb : Outport  VectorParamsAs1DForOutWhenUnconnected=off
  wires:
  HDL Counter1/1 -> Add/2, Multiport Switch/3, Relational Operator/1
  Relational Operator/1 -> Multiport Switch/1
  Constant/1 -> Relational Operator/2
  Add/1 -> Multiport Switch/2
  Constant1/1 -> Add/1
  Multiport Switch/1 -> Gain/1
  Gain2/1 -> Add5/1
  Add5/1 -> Abs1/1
  Constant6/1 -> Add5/2
  HDL Counter2/1 -> Gain2/1
  Abs1/1 -> Gain3/1
  Gain3/1 -> sanjb/1

== system yixiang/CBSVPWM/jxcbsv/siquah ==
  aH1 : Inport
  Constant2 : Constant  Value=0  OutDataTypeStr=int16  SampleTime=2e-8
  Data Type Conversion3 : DataTypeConversion  OutDataTypeStr=boolean  SaturateOnIntegerOverflow=off  RndMeth=Floor
  Data Type Conversion4 : DataTypeConversion  OutDataTypeStr=boolean  SaturateOnIntegerOverflow=off  RndMeth=Floor
  Logical Operator2 : Logic  Operator=NOT  AllPortsSameDT=off  OutDataTypeStr=boolean
  Switch3 : Switch  Threshold=15  SaturateOnIntegerOverflow=off  InputSameDT=off
  高电平计数 : hdlsllib/Sources/HDL Counter  CountType=Free running  CountInit=0  CountStep=1  CountMax=250  CountFromType=Initial value  CountFrom=0  CountResetPort=on  CountLoadPort=off  CountEnbPort=on  CountDirPort=off  CountHitOutputPort=off  CountDataType=Signed  CountWordLen=16  CountFracLen=0  CountSampTime=1
  ys : Outport
  wires:
  Data Type Conversion3/1 -> Logical Operator2/1
  aH1/1 -> Switch3/1, Data Type Conversion4/1, Data Type Conversion3/1
  Constant2/1 -> Switch3/3
  高电平计数/1 -> Switch3/2
  Logical Operator2/1 -> 高电平计数/1
  Data Type Conversion4/1 -> 高电平计数/2
  Switch3/1 -> ys/1

== system yixiang/CBSVPWM/jxcbsv/siquah1 ==
  aH1 : Inport
  Constant2 : Constant  Value=0  OutDataTypeStr=int16  SampleTime=2e-8
  Data Type Conversion3 : DataTypeConversion  OutDataTypeStr=boolean  SaturateOnIntegerOverflow=off  RndMeth=Floor
  Data Type Conversion4 : DataTypeConversion  OutDataTypeStr=boolean  SaturateOnIntegerOverflow=off  RndMeth=Floor
  Logical Operator2 : Logic  Operator=NOT  AllPortsSameDT=off  OutDataTypeStr=boolean
  Switch3 : Switch  Threshold=15  SaturateOnIntegerOverflow=off  InputSameDT=off
  高电平计数 : hdlsllib/Sources/HDL Counter  CountType=Free running  CountInit=0  CountStep=1  CountMax=250  CountFromType=Initial value  CountFrom=0  CountResetPort=on  CountLoadPort=off  CountEnbPort=on  CountDirPort=off  CountHitOutputPort=off  CountDataType=Signed  CountWordLen=16  CountFracLen=0  CountSampTime=1
  ys : Outport
  wires:
  Data Type Conversion3/1 -> Logical Operator2/1
  aH1/1 -> Switch3/1, Data Type Conversion4/1, Data Type Conversion3/1
  Constant2/1 -> Switch3/3
  高电平计数/1 -> Switch3/2
  Logical Operator2/1 -> 高电平计数/1
  Data Type Conversion4/1 -> 高电平计数/2
  Switch3/1 -> ys/1

== system yixiang/CBSVPWM/jxcbsv/siquah2 ==
  bH1 : Inport
  Constant2 : Constant  Value=0  OutDataTypeStr=int16  SampleTime=2e-8
  Data Type Conversion3 : DataTypeConversion  OutDataTypeStr=boolean  SaturateOnIntegerOverflow=off  RndMeth=Floor
  Data Type Conversion4 : DataTypeConversion  OutDataTypeStr=boolean  SaturateOnIntegerOverflow=off  RndMeth=Floor
  Logical Operator2 : Logic  Operator=NOT  AllPortsSameDT=off  OutDataTypeStr=boolean
  Switch3 : Switch  Threshold=15  SaturateOnIntegerOverflow=off  InputSameDT=off
  高电平计数 : hdlsllib/Sources/HDL Counter  CountType=Free running  CountInit=0  CountStep=1  CountMax=250  CountFromType=Initial value  CountFrom=0  CountResetPort=on  CountLoadPort=off  CountEnbPort=on  CountDirPort=off  CountHitOutputPort=off  CountDataType=Signed  CountWordLen=16  CountFracLen=0  CountSampTime=1
  ys : Outport
  wires:
  Data Type Conversion3/1 -> Logical Operator2/1
  bH1/1 -> Switch3/1, Data Type Conversion4/1, Data Type Conversion3/1
  Constant2/1 -> Switch3/3
  高电平计数/1 -> Switch3/2
  Logical Operator2/1 -> 高电平计数/1
  Data Type Conversion4/1 -> 高电平计数/2
  Switch3/1 -> ys/1

== system yixiang/CBSVPWM/jxcbsv/siquah3 ==
  cH1 : Inport
  Constant2 : Constant  Value=0  OutDataTypeStr=int16  SampleTime=2e-8
  Data Type Conversion3 : DataTypeConversion  OutDataTypeStr=boolean  SaturateOnIntegerOverflow=off  RndMeth=Floor
  Data Type Conversion4 : DataTypeConversion  OutDataTypeStr=boolean  SaturateOnIntegerOverflow=off  RndMeth=Floor
  Logical Operator2 : Logic  Operator=NOT  AllPortsSameDT=off  OutDataTypeStr=boolean
  Switch3 : Switch  Threshold=15  SaturateOnIntegerOverflow=off  InputSameDT=off
  高电平计数 : hdlsllib/Sources/HDL Counter  CountType=Free running  CountInit=0  CountStep=1  CountMax=250  CountFromType=Initial value  CountFrom=0  CountResetPort=on  CountLoadPort=off  CountEnbPort=on  CountDirPort=off  CountHitOutputPort=off  CountDataType=Signed  CountWordLen=16  CountFracLen=0  CountSampTime=1
  ys : Outport
  wires:
  Data Type Conversion3/1 -> Logical Operator2/1
  cH1/1 -> Switch3/1, Data Type Conversion4/1, Data Type Conversion3/1
  Constant2/1 -> Switch3/3
  高电平计数/1 -> Switch3/2
  Logical Operator2/1 -> 高电平计数/1
  Data Type Conversion4/1 -> 高电平计数/2
  Switch3/1 -> ys/1

== system yixiang/CBSVPWM/jxcbsv/siqual ==
  aL1 : Inport
  Constant2 : Constant  Value=0  OutDataTypeStr=int16  SampleTime=2e-8
  Data Type Conversion3 : DataTypeConversion  OutDataTypeStr=boolean  SaturateOnIntegerOverflow=off  RndMeth=Floor
  Data Type Conversion4 : DataTypeConversion  OutDataTypeStr=boolean  SaturateOnIntegerOverflow=off  RndMeth=Floor
  Logical Operator2 : Logic  Operator=NOT  AllPortsSameDT=off  OutDataTypeStr=boolean
  Switch3 : Switch  Threshold=15  SaturateOnIntegerOverflow=off  InputSameDT=off
  高电平计数 : hdlsllib/Sources/HDL Counter  CountType=Free running  CountInit=0  CountStep=1  CountMax=250  CountFromType=Initial value  CountFrom=0  CountResetPort=on  CountLoadPort=off  CountEnbPort=on  CountDirPort=off  CountHitOutputPort=off  CountDataType=Signed  CountWordLen=16  CountFracLen=0  CountSampTime=1
  ys : Outport
  wires:
  Data Type Conversion3/1 -> Logical Operator2/1
  aL1/1 -> Switch3/1, Data Type Conversion4/1, Data Type Conversion3/1
  Constant2/1 -> Switch3/3
  高电平计数/1 -> Switch3/2
  Logical Operator2/1 -> 高电平计数/1
  Data Type Conversion4/1 -> 高电平计数/2
  Switch3/1 -> ys/1

== system yixiang/CBSVPWM/jxcbsv/siqual1 ==
  aL1 : Inport
  Constant2 : Constant  Value=0  OutDataTypeStr=int16  SampleTime=2e-8
  Data Type Conversion3 : DataTypeConversion  OutDataTypeStr=boolean  SaturateOnIntegerOverflow=off  RndMeth=Floor
  Data Type Conversion4 : DataTypeConversion  OutDataTypeStr=boolean  SaturateOnIntegerOverflow=off  RndMeth=Floor
  Logical Operator2 : Logic  Operator=NOT  AllPortsSameDT=off  OutDataTypeStr=boolean
  Switch3 : Switch  Threshold=15  SaturateOnIntegerOverflow=off  InputSameDT=off
  高电平计数 : hdlsllib/Sources/HDL Counter  CountType=Free running  CountInit=0  CountStep=1  CountMax=250  CountFromType=Initial value  CountFrom=0  CountResetPort=on  CountLoadPort=off  CountEnbPort=on  CountDirPort=off  CountHitOutputPort=off  CountDataType=Signed  CountWordLen=16  CountFracLen=0  CountSampTime=1
  ys : Outport
  wires:
  Data Type Conversion3/1 -> Logical Operator2/1
  aL1/1 -> Switch3/1, Data Type Conversion4/1, Data Type Conversion3/1
  Constant2/1 -> Switch3/3
  高电平计数/1 -> Switch3/2
  Logical Operator2/1 -> 高电平计数/1
  Data Type Conversion4/1 -> 高电平计数/2
  Switch3/1 -> ys/1

== system yixiang/CBSVPWM/jxcbsv/siqual2 ==
  bL1 : Inport
  Constant2 : Constant  Value=0  OutDataTypeStr=int16  SampleTime=2e-8
  Data Type Conversion3 : DataTypeConversion  OutDataTypeStr=boolean  SaturateOnIntegerOverflow=off  RndMeth=Floor
  Data Type Conversion4 : DataTypeConversion  OutDataTypeStr=boolean  SaturateOnIntegerOverflow=off  RndMeth=Floor
  Logical Operator2 : Logic  Operator=NOT  AllPortsSameDT=off  OutDataTypeStr=boolean
  Switch3 : Switch  Threshold=15  SaturateOnIntegerOverflow=off  InputSameDT=off
  高电平计数 : hdlsllib/Sources/HDL Counter  CountType=Free running  CountInit=0  CountStep=1  CountMax=250  CountFromType=Initial value  CountFrom=0  CountResetPort=on  CountLoadPort=off  CountEnbPort=on  CountDirPort=off  CountHitOutputPort=off  CountDataType=Signed  CountWordLen=16  CountFracLen=0  CountSampTime=1
  ys : Outport
  wires:
  Data Type Conversion3/1 -> Logical Operator2/1
  bL1/1 -> Switch3/1, Data Type Conversion4/1, Data Type Conversion3/1
  Constant2/1 -> Switch3/3
  高电平计数/1 -> Switch3/2
  Logical Operator2/1 -> 高电平计数/1
  Data Type Conversion4/1 -> 高电平计数/2
  Switch3/1 -> ys/1

== system yixiang/CBSVPWM/jxcbsv/siqual3 ==
  cL1 : Inport
  Constant2 : Constant  Value=0  OutDataTypeStr=int16  SampleTime=2e-8
  Data Type Conversion3 : DataTypeConversion  OutDataTypeStr=boolean  SaturateOnIntegerOverflow=off  RndMeth=Floor
  Data Type Conversion4 : DataTypeConversion  OutDataTypeStr=boolean  SaturateOnIntegerOverflow=off  RndMeth=Floor
  Logical Operator2 : Logic  Operator=NOT  AllPortsSameDT=off  OutDataTypeStr=boolean
  Switch3 : Switch  Threshold=15  SaturateOnIntegerOverflow=off  InputSameDT=off
  高电平计数 : hdlsllib/Sources/HDL Counter  CountType=Free running  CountInit=0  CountStep=1  CountMax=250  CountFromType=Initial value  CountFrom=0  CountResetPort=on  CountLoadPort=off  CountEnbPort=on  CountDirPort=off  CountHitOutputPort=off  CountDataType=Signed  CountWordLen=16  CountFracLen=0  CountSampTime=1
  ys : Outport
  wires:
  Data Type Conversion3/1 -> Logical Operator2/1
  cL1/1 -> Switch3/1, Data Type Conversion4/1, Data Type Conversion3/1
  Constant2/1 -> Switch3/3
  高电平计数/1 -> Switch3/2
  Logical Operator2/1 -> 高电平计数/1
  Data Type Conversion4/1 -> 高电平计数/2
  Switch3/1 -> ys/1

== system yixiang/CBSVPWM/jxcbsv/siqubh ==
  bH1 : Inport
  Constant2 : Constant  Value=0  OutDataTypeStr=int16  SampleTime=2e-8
  Data Type Conversion3 : DataTypeConversion  OutDataTypeStr=boolean  SaturateOnIntegerOverflow=off  RndMeth=Floor
  Data Type Conversion4 : DataTypeConversion  OutDataTypeStr=boolean  SaturateOnIntegerOverflow=off  RndMeth=Floor
  Logical Operator2 : Logic  Operator=NOT  AllPortsSameDT=off  OutDataTypeStr=boolean
  Switch3 : Switch  Threshold=15  SaturateOnIntegerOverflow=off  InputSameDT=off
  高电平计数 : hdlsllib/Sources/HDL Counter  CountType=Free running  CountInit=0  CountStep=1  CountMax=250  CountFromType=Initial value  CountFrom=0  CountResetPort=on  CountLoadPort=off  CountEnbPort=on  CountDirPort=off  CountHitOutputPort=off  CountDataType=Signed  CountWordLen=16  CountFracLen=0  CountSampTime=1
  ys : Outport
  wires:
  Data Type Conversion3/1 -> Logical Operator2/1
  bH1/1 -> Switch3/1, Data Type Conversion4/1, Data Type Conversion3/1
  Constant2/1 -> Switch3/3
  高电平计数/1 -> Switch3/2
  Logical Operator2/1 -> 高电平计数/1
  Data Type Conversion4/1 -> 高电平计数/2
  Switch3/1 -> ys/1

== system yixiang/CBSVPWM/jxcbsv/siqubl ==
  bL1 : Inport
  Constant2 : Constant  Value=0  OutDataTypeStr=int16  SampleTime=2e-8
  Data Type Conversion3 : DataTypeConversion  OutDataTypeStr=boolean  SaturateOnIntegerOverflow=off  RndMeth=Floor
  Data Type Conversion4 : DataTypeConversion  OutDataTypeStr=boolean  SaturateOnIntegerOverflow=off  RndMeth=Floor
  Logical Operator2 : Logic  Operator=NOT  AllPortsSameDT=off  OutDataTypeStr=boolean
  Switch3 : Switch  Threshold=15  SaturateOnIntegerOverflow=off  InputSameDT=off
  高电平计数 : hdlsllib/Sources/HDL Counter  CountType=Free running  CountInit=0  CountStep=1  CountMax=250  CountFromType=Initial value  CountFrom=0  CountResetPort=on  CountLoadPort=off  CountEnbPort=on  CountDirPort=off  CountHitOutputPort=off  CountDataType=Signed  CountWordLen=16  CountFracLen=0  CountSampTime=1
  ys : Outport
  wires:
  Data Type Conversion3/1 -> Logical Operator2/1
  bL1/1 -> Switch3/1, Data Type Conversion4/1, Data Type Conversion3/1
  Constant2/1 -> Switch3/3
  高电平计数/1 -> Switch3/2
  Logical Operator2/1 -> 高电平计数/1
  Data Type Conversion4/1 -> 高电平计数/2
  Switch3/1 -> ys/1

== system yixiang/CBSVPWM/jxcbsv/siquch ==
  cH1 : Inport
  Constant2 : Constant  Value=0  OutDataTypeStr=int16  SampleTime=2e-8
  Data Type Conversion3 : DataTypeConversion  OutDataTypeStr=boolean  SaturateOnIntegerOverflow=off  RndMeth=Floor
  Data Type Conversion4 : DataTypeConversion  OutDataTypeStr=boolean  SaturateOnIntegerOverflow=off  RndMeth=Floor
  Logical Operator2 : Logic  Operator=NOT  AllPortsSameDT=off  OutDataTypeStr=boolean
  Switch3 : Switch  Threshold=15  SaturateOnIntegerOverflow=off  InputSameDT=off
  高电平计数 : hdlsllib/Sources/HDL Counter  CountType=Free running  CountInit=0  CountStep=1  CountMax=250  CountFromType=Initial value  CountFrom=0  CountResetPort=on  CountLoadPort=off  CountEnbPort=on  CountDirPort=off  CountHitOutputPort=off  CountDataType=Signed  CountWordLen=16  CountFracLen=0  CountSampTime=1
  ys : Outport
  wires:
  Data Type Conversion3/1 -> Logical Operator2/1
  cH1/1 -> Switch3/1, Data Type Conversion4/1, Data Type Conversion3/1
  Constant2/1 -> Switch3/3
  高电平计数/1 -> Switch3/2
  Logical Operator2/1 -> 高电平计数/1
  Data Type Conversion4/1 -> 高电平计数/2
  Switch3/1 -> ys/1

== system yixiang/CBSVPWM/jxcbsv/siqucl ==
  cL1 : Inport
  Constant2 : Constant  Value=0  OutDataTypeStr=int16  SampleTime=2e-8
  Data Type Conversion3 : DataTypeConversion  OutDataTypeStr=boolean  SaturateOnIntegerOverflow=off  RndMeth=Floor
  Data Type Conversion4 : DataTypeConversion  OutDataTypeStr=boolean  SaturateOnIntegerOverflow=off  RndMeth=Floor
  Logical Operator2 : Logic  Operator=NOT  AllPortsSameDT=off  OutDataTypeStr=boolean
  Switch3 : Switch  Threshold=15  SaturateOnIntegerOverflow=off  InputSameDT=off
  高电平计数 : hdlsllib/Sources/HDL Counter  CountType=Free running  CountInit=0  CountStep=1  CountMax=250  CountFromType=Initial value  CountFrom=0  CountResetPort=on  CountLoadPort=off  CountEnbPort=on  CountDirPort=off  CountHitOutputPort=off  CountDataType=Signed  CountWordLen=16  CountFracLen=0  CountSampTime=1
  ys : Outport
  wires:
  Data Type Conversion3/1 -> Logical Operator2/1
  cL1/1 -> Switch3/1, Data Type Conversion4/1, Data Type Conversion3/1
  Constant2/1 -> Switch3/3
  高电平计数/1 -> Switch3/2
  Logical Operator2/1 -> 高电平计数/1
  Data Type Conversion4/1 -> 高电平计数/2
  Switch3/1 -> ys/1

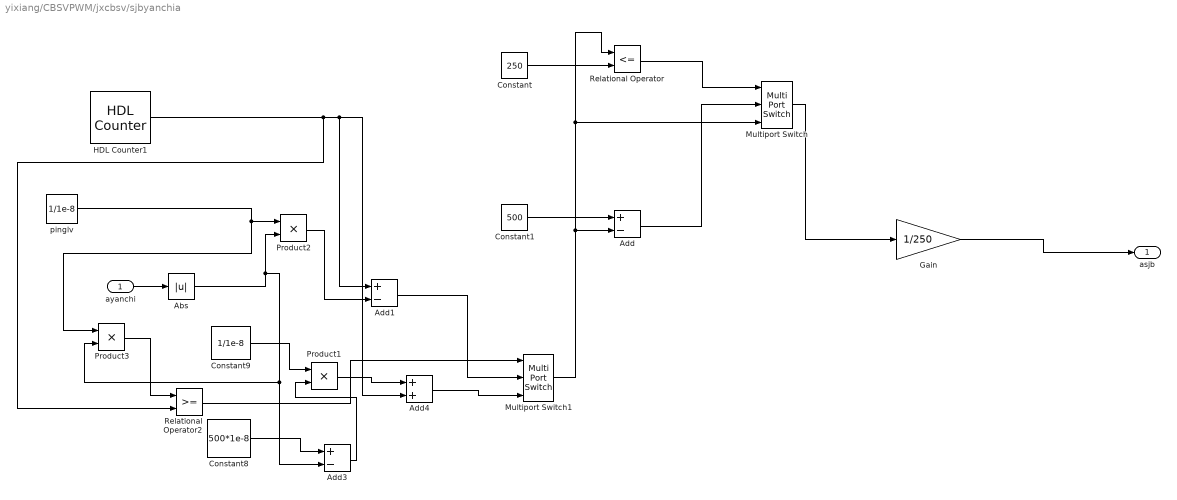
== system yixiang/CBSVPWM/jxcbsv/sjbyanchia ==
  ayanchi : Inport
  Abs : Abs  SaturateOnIntegerOverflow=off
  Add : Sum  Inputs=+-
  Add1 : Sum  Inputs=+-
  Add3 : Sum  Inputs=+-  OutDataTypeStr=fixdt(1,30,29)  AccumDataTypeStr=fixdt(1,30,29)
  Add4 : Sum
  Constant : Constant  Value=250  OutDataTypeStr=fixdt(1,20,0)  SampleTime=1e-8
  Constant1 : Constant  Value=500  OutDataTypeStr=fixdt(1,20,0)  SampleTime=1e-8
  Constant8 : Constant  Value=500*1e-8  OutDataTypeStr=fixdt(1,23,22)  SampleTime=1e-8
  Constant9 : Constant  Value=1/1e-8  OutDataTypeStr=fixdt(1,28,0)  SampleTime=1e-8
  Gain : Gain  Gain=1/250  OutDataTypeStr=fixdt(1,20,18)
  HDL Counter1 : hdlsllib/Sources/HDL Counter  CountType=Count limited  CountInit=0  CountStep=1  CountMax=500  CountFromType=Initial value  CountFrom=0  CountResetPort=off  CountLoadPort=off  CountEnbPort=off  CountDirPort=off  CountHitOutputPort=off  CountDataType=Unsigned  CountWordLen=32  CountFracLen=0  CountSampTime=1/10000/10000
  Multiport Switch : MultiPortSwitch  DataPortOrder=Zero-based contiguous  Inputs=2  zeroidx=on  OutDataTypeStr=fixdt(1,20,0)  SaturateOnIntegerOverflow=off  InputSameDT=off
  Multiport Switch1 : MultiPortSwitch  DataPortOrder=Zero-based contiguous  Inputs=2  zeroidx=on  OutDataTypeStr=fixdt(1,20,0)  SaturateOnIntegerOverflow=off  InputSameDT=off
  Product1 : Product  OutDataTypeStr=int16
  Product2 : Product  OutDataTypeStr=int32
  Product3 : Product  OutDataTypeStr=int16
  Relational Operator : RelationalOperator  Operator=<=  OutDataTypeStr=boolean  InputSameDT=off
  Relational Operator2 : RelationalOperator  OutDataTypeStr=boolean  InputSameDT=off
  pinglv : Constant  Value=1/1e-8  OutDataTypeStr=fixdt(1,32,0)  SampleTime=1e-8
  asjb : Outport
  wires:
  Relational Operator/1 -> Multiport Switch/1
  pinglv/1 -> Product3/1, Product2/1
  Product1/1 -> Add4/1
  Add1/1 -> Multiport Switch1/2
  Multiport Switch/1 -> Gain/1
  Constant9/1 -> Product1/1
  Relational Operator2/1 -> Multiport Switch1/1
  Product3/1 -> Relational Operator2/1
  ayanchi/1 -> Abs/1
  Add/1 -> Multiport Switch/2
  Add4/1 -> Multiport Switch1/3
  Constant8/1 -> Add3/1
  Add3/1 -> Product1/2
  Multiport Switch1/1 -> Relational Operator/1, Multiport Switch/3, Add/2
  HDL Counter1/1 -> Relational Operator2/2, Add4/2, Add1/1
  Constant1/1 -> Add/1
  Product2/1 -> Add1/2
  Constant/1 -> Relational Operator/2
  Gain/1 -> asjb/1
  Abs/1 -> Product2/2, Product3/2, Add3/2

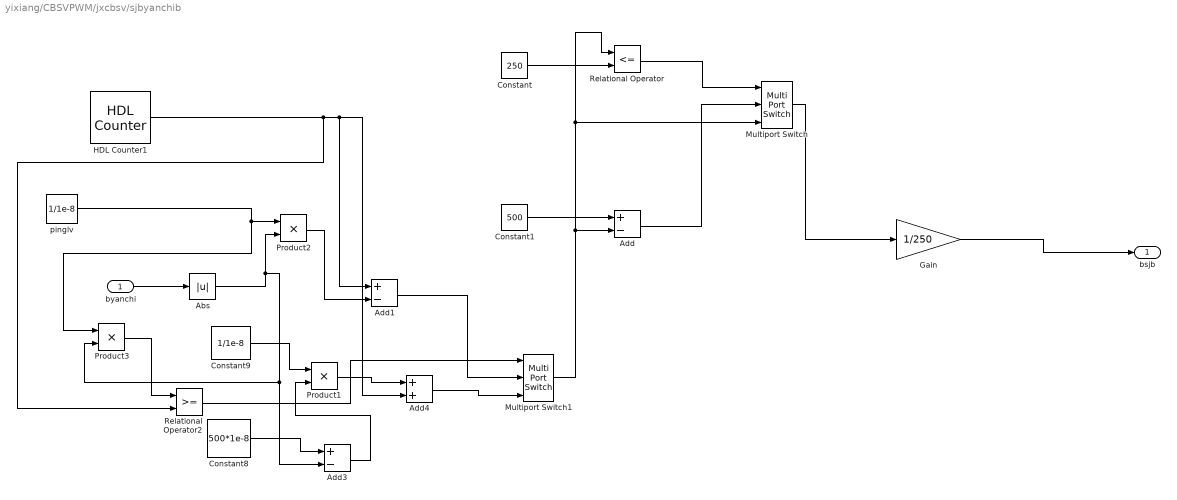
== system yixiang/CBSVPWM/jxcbsv/sjbyanchib ==
  byanchi : Inport
  Abs : Abs  SaturateOnIntegerOverflow=off
  Add : Sum  Inputs=+-
  Add1 : Sum  Inputs=+-
  Add3 : Sum  Inputs=+-  OutDataTypeStr=fixdt(1,30,29)  AccumDataTypeStr=fixdt(1,30,29)
  Add4 : Sum
  Constant : Constant  Value=250  OutDataTypeStr=fixdt(1,20,0)  SampleTime=1e-8
  Constant1 : Constant  Value=500  OutDataTypeStr=fixdt(1,20,0)  SampleTime=1e-8
  Constant8 : Constant  Value=500*1e-8  OutDataTypeStr=fixdt(1,23,22)  SampleTime=1e-8
  Constant9 : Constant  Value=1/1e-8  OutDataTypeStr=fixdt(1,28,0)  SampleTime=1e-8
  Gain : Gain  Gain=1/250  OutDataTypeStr=fixdt(1,20,18)
  HDL Counter1 : hdlsllib/Sources/HDL Counter  CountType=Count limited  CountInit=0  CountStep=1  CountMax=500  CountFromType=Initial value  CountFrom=0  CountResetPort=off  CountLoadPort=off  CountEnbPort=off  CountDirPort=off  CountHitOutputPort=off  CountDataType=Unsigned  CountWordLen=20  CountFracLen=0  CountSampTime=1/10000/10000
  Multiport Switch : MultiPortSwitch  DataPortOrder=Zero-based contiguous  Inputs=2  zeroidx=on  OutDataTypeStr=fixdt(1,20,0)  SaturateOnIntegerOverflow=off  InputSameDT=off
  Multiport Switch1 : MultiPortSwitch  DataPortOrder=Zero-based contiguous  Inputs=2  zeroidx=on  OutDataTypeStr=fixdt(1,20,0)  SaturateOnIntegerOverflow=off  InputSameDT=off
  Product1 : Product  OutDataTypeStr=int16
  Product2 : Product  OutDataTypeStr=int16
  Product3 : Product  OutDataTypeStr=int16
  Relational Operator : RelationalOperator  Operator=<=  OutDataTypeStr=boolean  InputSameDT=off
  Relational Operator2 : RelationalOperator  OutDataTypeStr=boolean  InputSameDT=off
  pinglv : Constant  Value=1/1e-8  OutDataTypeStr=fixdt(1,28,0)  SampleTime=1e-8
  bsjb : Outport
  wires:
  Relational Operator/1 -> Multiport Switch/1
  pinglv/1 -> Product3/1, Product2/1
  Product1/1 -> Add4/1
  Add1/1 -> Multiport Switch1/2
  Multiport Switch/1 -> Gain/1
  Constant9/1 -> Product1/1
  Relational Operator2/1 -> Multiport Switch1/1
  Product3/1 -> Relational Operator2/1
  byanchi/1 -> Abs/1
  Add/1 -> Multiport Switch/2
  Add4/1 -> Multiport Switch1/3
  Constant8/1 -> Add3/1
  Add3/1 -> Product1/2
  Multiport Switch1/1 -> Relational Operator/1, Multiport Switch/3, Add/2
  HDL Counter1/1 -> Relational Operator2/2, Add4/2, Add1/1
  Constant1/1 -> Add/1
  Product2/1 -> Add1/2
  Constant/1 -> Relational Operator/2
  Gain/1 -> bsjb/1
  Abs/1 -> Product2/2, Product3/2, Add3/2

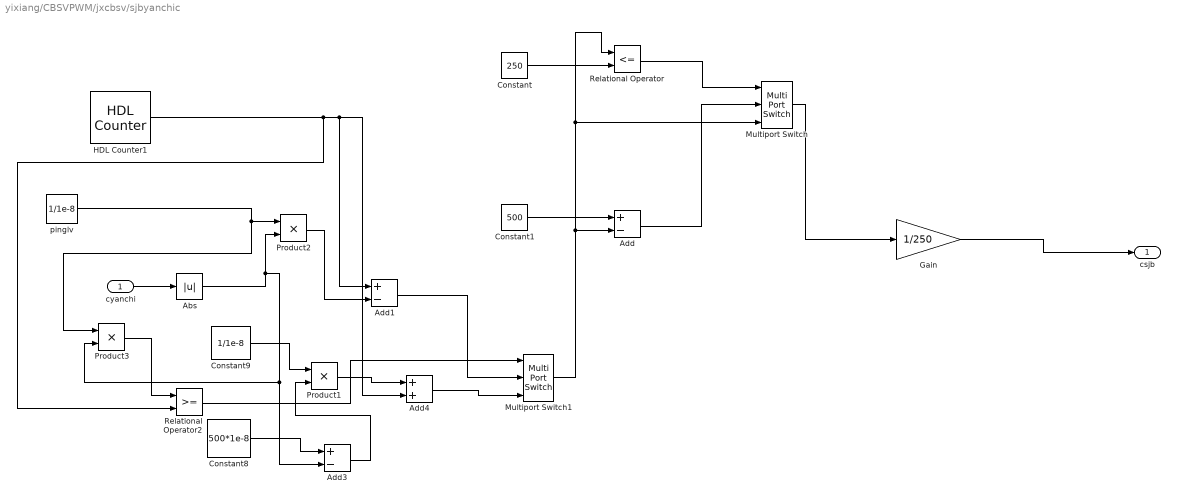
== system yixiang/CBSVPWM/jxcbsv/sjbyanchic ==
  cyanchi : Inport
  Abs : Abs  SaturateOnIntegerOverflow=off
  Add : Sum  Inputs=+-
  Add1 : Sum  Inputs=+-
  Add3 : Sum  Inputs=+-  OutDataTypeStr=fixdt(1,30,29)  AccumDataTypeStr=fixdt(1,30,29)
  Add4 : Sum
  Constant : Constant  Value=250  OutDataTypeStr=fixdt(1,20,0)  SampleTime=1e-8
  Constant1 : Constant  Value=500  OutDataTypeStr=fixdt(1,20,0)  SampleTime=1e-8
  Constant8 : Constant  Value=500*1e-8  OutDataTypeStr=fixdt(1,23,22)  SampleTime=1e-8
  Constant9 : Constant  Value=1/1e-8  OutDataTypeStr=fixdt(1,28,0)  SampleTime=1e-8
  Gain : Gain  Gain=1/250  OutDataTypeStr=fixdt(1,20,18)
  HDL Counter1 : hdlsllib/Sources/HDL Counter  CountType=Count limited  CountInit=0  CountStep=1  CountMax=500  CountFromType=Initial value  CountFrom=0  CountResetPort=off  CountLoadPort=off  CountEnbPort=off  CountDirPort=off  CountHitOutputPort=off  CountDataType=Unsigned  CountWordLen=20  CountFracLen=0  CountSampTime=1/10000/10000
  Multiport Switch : MultiPortSwitch  DataPortOrder=Zero-based contiguous  Inputs=2  zeroidx=on  OutDataTypeStr=fixdt(1,20,0)  SaturateOnIntegerOverflow=off  InputSameDT=off
  Multiport Switch1 : MultiPortSwitch  DataPortOrder=Zero-based contiguous  Inputs=2  zeroidx=on  OutDataTypeStr=fixdt(1,20,0)  SaturateOnIntegerOverflow=off  InputSameDT=off
  Product1 : Product  OutDataTypeStr=int16
  Product2 : Product  OutDataTypeStr=int16
  Product3 : Product  OutDataTypeStr=int16
  Relational Operator : RelationalOperator  Operator=<=  OutDataTypeStr=boolean  InputSameDT=off
  Relational Operator2 : RelationalOperator  OutDataTypeStr=boolean  InputSameDT=off
  pinglv : Constant  Value=1/1e-8  OutDataTypeStr=fixdt(1,28,0)  SampleTime=1e-8
  csjb : Outport
  wires:
  Relational Operator/1 -> Multiport Switch/1
  pinglv/1 -> Product3/1, Product2/1
  Product1/1 -> Add4/1
  Add1/1 -> Multiport Switch1/2
  Multiport Switch/1 -> Gain/1
  Constant9/1 -> Product1/1
  Relational Operator2/1 -> Multiport Switch1/1
  Product3/1 -> Relational Operator2/1
  cyanchi/1 -> Abs/1
  Add/1 -> Multiport Switch/2
  Add4/1 -> Multiport Switch1/3
  Constant8/1 -> Add3/1
  Add3/1 -> Product1/2
  Multiport Switch1/1 -> Relational Operator/1, Multiport Switch/3, Add/2
  HDL Counter1/1 -> Relational Operator2/2, Add4/2, Add1/1
  Constant1/1 -> Add/1
  Product2/1 -> Add1/2
  Constant/1 -> Relational Operator/2
  Gain/1 -> csjb/1
  Abs/1 -> Product2/2, Product3/2, Add3/2

== system yixiang/CBSVPWM/jxcbsv/yixiang2 ==
  bH1 : Inport
  zmc1 : Subsystem
  zmcxc6 : Subsystem
  bHyan : Outport
  wires:
  zmcxc6/1(aL1) -> bHyan/1
  zmc1/1(bH1) -> zmcxc6/1(bH1)
  bH1/1 -> zmc1/1(aH1)

== system yixiang/CBSVPWM/jxcbsv/yixiang4 ==
  cH1 : Inport
  zmc1 : Subsystem
  zmcxc6 : Subsystem
  cHyan : Outport
  wires:
  zmcxc6/1(aL1) -> cHyan/1
  zmc1/1(bH1) -> zmcxc6/1(bH1)
  cH1/1 -> zmc1/1(aH1)

== system yixiang/CBSVPWM/jxcbsv/yixiang5 ==
  cH1 : Inport
  zmc1 : Subsystem
  zmcxc6 : Subsystem
  cHyan : Outport
  wires:
  zmcxc6/1(aL1) -> cHyan/1
  zmc1/1(bH1) -> zmcxc6/1(bH1)
  cH1/1 -> zmc1/1(aH1)
